simulink model "CLIK_inv_jacob_1order"  (R2021a)
settings: Solver=VariableStepAuto  StartTime=0.0  StopTime=50  MaxStep=1e-3  RelTol=1e-3
values from neighbouring files (symbols this model uses):
  K = diag([1000 10 100])    [pseudo_traiettoria.m]
  q0 = scara.ikine(T0, 'mask', [1 1 1 1 0 0])    [pseudo_traiettoria.m]    (also in traiettoria.m)
  Tc = 0.001    [pseudo_traiettoria.m]    (also in traiettoria.m)
undefined symbols (not defined in the file or in its folder): DiscIntNeverNeededParam
settings Model: Creator=ciro  LastModifiedBy=Ciro

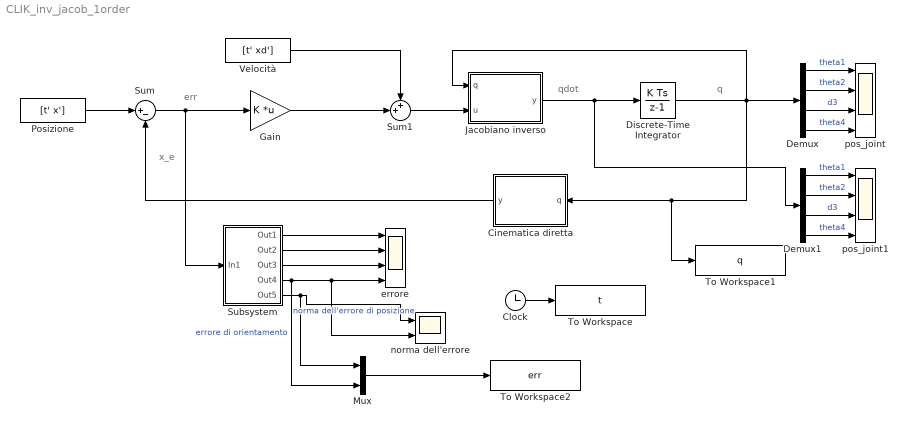
== system CLIK_inv_jacob_1order ==
  note: x_e
  note: err
  note: q
  note: qdot
  Cinematica diretta : MATLAB Function  TreatAsAtomicUnit=on
  Clock : Clock
  Demux : Demux
  Demux1 : Demux
  Discrete-Time Integrator : DiscreteIntegrator  InitialCondition=q0  SampleTime=Tc  ICPrevOutput=DiscIntNeverNeededParam  ICPrevScaledInput=DiscIntNeverNeededParam
  Gain : Gain  Gain=K  Multiplication=Matrix(K*u)
  Jacobiano inverso : MATLAB Function  TreatAsAtomicUnit=on
  Mux : Mux  Inputs=2
  Posizione : FromWorkspace  VariableName=[t' x']  SampleTime=Tc  OutputAfterFinalValue=Holding final value
  Subsystem : Subsystem
  Sum : Sum  Inputs=|+-
  Sum1 : Sum  Inputs=++|
  To Workspace : ToWorkspace  VariableName=t  SampleTime=-1
      settings: Save2DSignal=2-D array (concatenate along first dimension)
  To Workspace1 : ToWorkspace  VariableName=q  SampleTime=-1
      settings: Save2DSignal=2-D array (concatenate along first dimension)
  To Workspace2 : ToWorkspace  VariableName=err  SampleTime=-1
      settings: Save2DSignal=2-D array (concatenate along first dimension)
  Velocità : FromWorkspace  VariableName=[t' xd']  SampleTime=Tc  OutputAfterFinalValue=Holding final value
  errore : Scope  NumInputPorts=4
  norma dell'errore : Scope  NumInputPorts=2
  pos_joint : Scope  NumInputPorts=4
  pos_joint1 : Scope  NumInputPorts=4
  wires:
  Posizione/1 -> Sum/1
  Sum1/1 -> Jacobiano inverso/2(u)
  Cinematica diretta/1(y) -> Sum/2
  Demux/1 -> pos_joint/1  "theta1"
  Demux/2 -> pos_joint/2  "theta2"
  Demux/3 -> pos_joint/3  "d3"
  Demux/4 -> pos_joint/4  "theta4"
  Sum/1 -> Gain/1, Subsystem/1(In1)
  Subsystem/4(Out4) -> Mux/2, norma dell'errore/2, errore/4  "errore di orientamento"
  Subsystem/1(Out1) -> errore/1
  Subsystem/2(Out2) -> errore/2
  Subsystem/3(Out3) -> errore/3
  Subsystem/5(Out5) -> Mux/1, norma dell'errore/1  "norma dell'errore di posizione"
  Gain/1 -> Sum1/2
  Velocità/1 -> Sum1/1
  Clock/1 -> To Workspace/1
  Discrete-Time Integrator/1 -> To Workspace1/1, Cinematica diretta/1(q), Demux/1, Jacobiano inverso/1(q)
  Jacobiano inverso/1(y) -> Demux1/1, Discrete-Time Integrator/1
  Demux1/4 -> pos_joint1/4  "theta4"
  Demux1/3 -> pos_joint1/3  "d3"
  Demux1/2 -> pos_joint1/2  "theta2"
  Demux1/1 -> pos_joint1/1  "theta1"
  Mux/1 -> To Workspace2/1

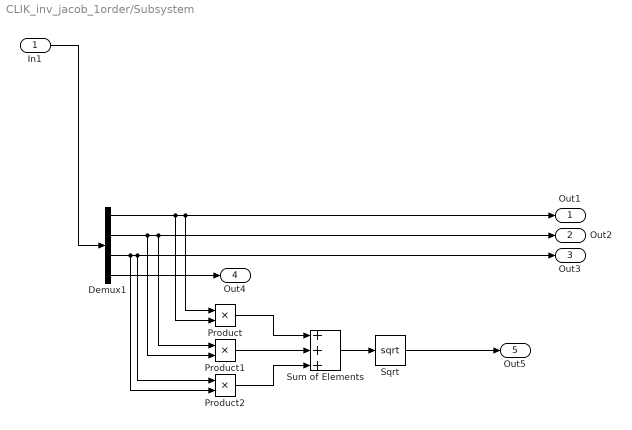
== system CLIK_inv_jacob_1order/Subsystem ==
  In1 : Inport
  Demux1 : Demux
  Product : Product
  Product1 : Product
  Product2 : Product
  Sqrt : Sqrt  SaturateOnIntegerOverflow=on
  Sum of Elements : Sum  Inputs=+++
  Out1 : Outport
  Out2 : Outport  Port=2
  Out3 : Outport  Port=3
  Out4 : Outport  Port=4
  Out5 : Outport  Port=5
  wires:
  Demux1/3 -> Product2/2, Out3/1, Product2/1
  Demux1/2 -> Product1/2, Out2/1, Product1/1
  Product/1 -> Sum of Elements/1
  Sum of Elements/1 -> Sqrt/1
  Product1/1 -> Sum of Elements/2
  Demux1/4 -> Out4/1
  Demux1/1 -> Product/2, Out1/1, Product/1
  Product2/1 -> Sum of Elements/3
  Sqrt/1 -> Out5/1
  In1/1 -> Demux1/1

== matlab function CLIK_inv_jacob_1order/Jacobiano inverso ==
  data: q input; u input; y output
function y = fcn(q, u)

J = [ -0.5*(sin(q(1))+sin(q(1)+q(2))) -0.5*sin(q(1)+q(2))  0  0;
       0.5*(cos(q(1))+cos(q(1)+q(2)))  0.5*cos(q(1)+q(2))  0  0;
       0                               0                  -1  0;
       1                               1                   0 -1];

y = J\u;

== matlab function CLIK_inv_jacob_1order/Cinematica diretta ==
  data: q input; y output
function y = fcn(q)

xe = [0.5*(cos(q(1))+cos(q(1)+q(2)));
      0.5*(sin(q(1))+sin(q(1)+q(2)));
      0.8-q(3);
      q(1)+q(2)-q(4)];

y = xe;
